simulink model "whole_system"  (R2016a)
settings: Solver=VariableStepAuto  StartTime=0.0  StopTime=0.25*100e6  RelTol=1e-3
libraries: xbsIndex_r4 x92, powerlib_meascontrol x4
settings Model: Creator=Jorge  LastModifiedBy=Jorge

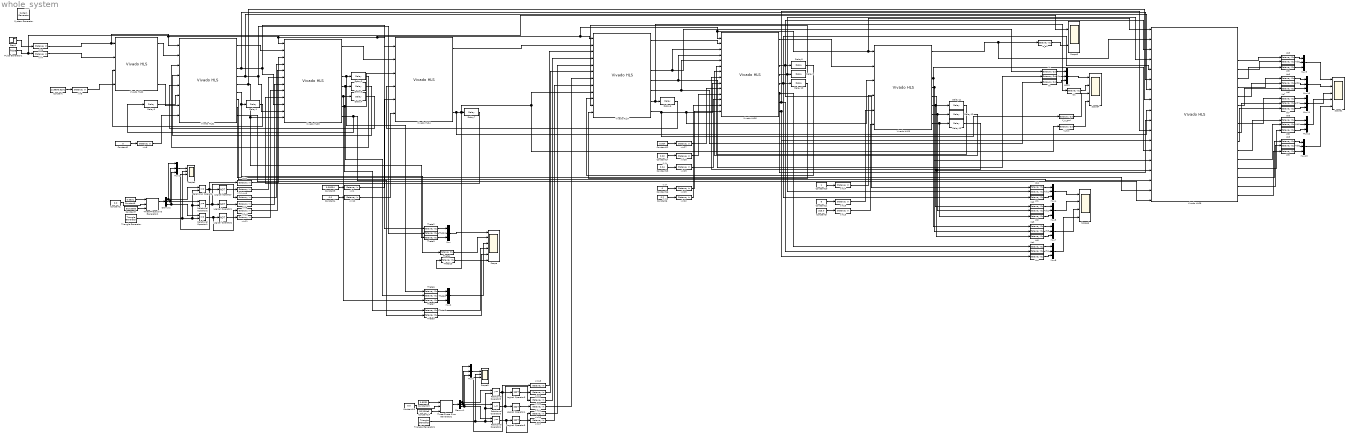
== system whole_system ==
  note: 0.04
  note: 0.04
  note: 0.04
  " System Generator" : xbsIndex_r4/ System Generator  Tag=genX  xilinxfamily=zynq  part=xc7z020  speed=-1  package=clg400  synthesis_tool=Vivado  clock_wrapper=Clock Enables  directory=./netlist  proj_type=Vivado  Synth_file=Vivado Synthesis Defaults  Impl_file=Vivado Implementation Defaults  testbench=off  simulink_period=1  sysclk_period=10  dcm_input_clock_period=10  incr_netlist=off  trim_vbits=Everywhere in SubSystem  dbl_ovrd=According to Block Masks  core_generation=According to Block Masks  run_coregen=off  deprecated_control=off  eval_field=0  block_type=sysgen
  Constant : Constant  Value=119856.8291
  Constant1 : Constant  Value=0.0
  Constant10 : Constant
  Constant11 : Constant  Value=8
  Constant12 : Constant  Value=0.004
  Constant13 : Constant  Value=0.0
  Constant14 : Constant  Value=50/100e6
  Constant16 : Constant  Value=0
  Constant17 : Constant  Value=0.02
  Constant18 : Constant  Value=0.04
  Constant19 : Constant  Value=0.6531
  Constant2 : Constant  Value=0
  Constant3 : Constant  Value=0.00004
  Constant4 : Constant  Value=0.0
  Constant5 : Constant  Value=325.0
  Constant6 : Constant  Value=0.5
  Constant7 : Constant  Value=50/100e6
  Constant8 : Constant  Value=0.6531
  Delay{1..13} (13 alike) : xbsIndex_r4/Delay  rst=off  infoeditControl=Selection of Reset will increase slice count due to use of real FFs and instead of SRLs  en=off  latency=1  reg_retiming=off  dbl_ovrd=off  block_type=delay
  Demux1 : Demux  Outputs=3
  Demux2 : Demux  Outputs=3
  Idc : xbsIndex_r4/Gateway Out  inherit_from_input=off  hdl_port=on  rows=1  columns=1  UseAsDAC=off  DACChannel='1'  interface=None  automatic_assignment=on  address_offset=hex2dec('00')  intf_name=''  intf_description=''  timing_constraint=None  locs_specified=off  LOCs={}  io_standard={}  block_type=gatewayout
  Is_a2 : xbsIndex_r4/Gateway Out  inherit_from_input=off  hdl_port=on  rows=1  columns=1  UseAsDAC=off  DACChannel='1'  interface=None  automatic_assignment=on  address_offset=hex2dec('00')  intf_name=''  intf_description=''  timing_constraint=None  locs_specified=off  LOCs={}  io_standard={}  block_type=gatewayout
  Logical Operator{,1..5} (6 alike) : Logic  Operator=NOT  AllPortsSameDT=off  OutDataTypeStr=boolean
  Mux{,1..13} (14 alike) : Mux  Inputs=3
  Pulse Generator1 : DiscretePulseGenerator  PulseType=Time based  Period=200  PulseWidth=50
  Relational Operator{,1..5} (6 alike) : RelationalOperator  OutDataTypeStr=boolean  ZeroCross=off
  Scope : Scope  NumInputPorts=6
  Scope1 : Scope  NumInputPorts=5
  Scope{2,4..6} (4 alike) : Scope  NumInputPorts=4
  Scope3 : Scope  NumInputPorts=2
  Step1 : Step  Time=1e-6  SampleTime=0
  Theta{1..10} (10 alike) : xbsIndex_r4/Gateway Out  inherit_from_input=off  hdl_port=on  rows=1  columns=1  UseAsDAC=off  DACChannel='1'  interface=None  automatic_assignment=on  address_offset=hex2dec('00')  intf_name=''  intf_description=''  timing_constraint=None  locs_specified=off  LOCs={}  io_standard={}  block_type=gatewayout
  Three-Phase Sine Generator1 : powerlib_meascontrol/Pulse & Signal Generators/Three-Phase Sine Generator  Ts=1
  Three-Phase Sine Generator2 : powerlib_meascontrol/Pulse & Signal Generators/Three-Phase Sine Generator  Ts=1
  Triangle Generator : powerlib_meascontrol/Pulse & Signal Generators/Triangle Generator  Freq=5e3/100e6  Phase=0  Ts=1
  Triangle Generator1 : powerlib_meascontrol/Pulse & Signal Generators/Triangle Generator  Freq=5e3/100e6  Phase=0  Ts=1
  V_bus : xbsIndex_r4/Gateway Out  inherit_from_input=off  hdl_port=on  rows=1  columns=1  UseAsDAC=off  DACChannel='1'  interface=None  automatic_assignment=on  address_offset=hex2dec('00')  intf_name=''  intf_description=''  timing_constraint=None  locs_specified=off  LOCs={}  io_standard={}  block_type=gatewayout
  V_n_gnd : xbsIndex_r4/Gateway Out  inherit_from_input=off  hdl_port=on  rows=1  columns=1  UseAsDAC=off  DACChannel='1'  interface=None  automatic_assignment=on  address_offset=hex2dec('00')  intf_name=''  intf_description=''  timing_constraint=None  locs_specified=off  LOCs={}  io_standard={}  block_type=gatewayout
  Va{,1..9} (10 alike) : xbsIndex_r4/Gateway Out  inherit_from_input=off  hdl_port=on  rows=1  columns=1  UseAsDAC=off  DACChannel='1'  interface=None  automatic_assignment=on  address_offset=hex2dec('00')  intf_name=''  intf_description=''  timing_constraint=None  locs_specified=off  LOCs={}  io_standard={}  block_type=gatewayout
  Vb{,1..9} (10 alike) : xbsIndex_r4/Gateway Out  inherit_from_input=off  hdl_port=on  rows=1  columns=1  UseAsDAC=off  DACChannel='1'  interface=None  automatic_assignment=on  address_offset=hex2dec('00')  intf_name=''  intf_description=''  timing_constraint=None  locs_specified=off  LOCs={}  io_standard={}  block_type=gatewayout
  Vc{,1..9} (10 alike) : xbsIndex_r4/Gateway Out  inherit_from_input=off  hdl_port=on  rows=1  columns=1  UseAsDAC=off  DACChannel='1'  interface=None  automatic_assignment=on  address_offset=hex2dec('00')  intf_name=''  intf_description=''  timing_constraint=None  locs_specified=off  LOCs={}  io_standard={}  block_type=gatewayout
  Vivado HLS1 : xbsIndex_r4/Vivado HLS  anytable='C:/Users/Jorge/Documents/GitHub/nvHIL/hls/pmsm_V2/pmsm_V2_prj/sol_sysgen'  fast_sim=off  display_datatype=on  rate_propagation_method=Simulink system period  model_file_path=''  latency=1  block_type=hls
      settings: infoedit=This block allows including C,C++ and SystemC source files in System Generator for DSP designs.
  Vivado HLS2 : xbsIndex_r4/Vivado HLS  anytable='C:\Users\Jorge\Documents\GitHub\nvHIL\hls\wind_tur_V2\wind_turb_V2_prj\sol_sysgen'  fast_sim=off  display_datatype=on  rate_propagation_method=Simulink system period  model_file_path=''  latency=1  block_type=hls
      settings: infoedit=This block allows including C,C++ and SystemC source files in System Generator for DSP designs.
  Vivado HLS3 : xbsIndex_r4/Vivado HLS  anytable='C:\Users\Jorge\Documents\GitHub\nvHIL\hls\pmsm_3ph_inv_V2\pmsm_inv_prj\sol_sysgen'  fast_sim=off  display_datatype=on  rate_propagation_method=Simulink system period  model_file_path=''  latency=1  block_type=hls
      settings: infoedit=This block allows including C,C++ and SystemC source files in System Generator for DSP designs.
  Vivado HLS4 : xbsIndex_r4/Vivado HLS  anytable='C:\Users\Jorge\Documents\GitHub\nvHIL\hls\DC_bus_V2\dc_bus_prj\sol_sysgen'  fast_sim=off  display_datatype=on  rate_propagation_method=Simulink system period  model_file_path=''  latency=1  block_type=hls
      settings: infoedit=This block allows including C,C++ and SystemC source files in System Generator for DSP designs.
  Vivado HLS5 : xbsIndex_r4/Vivado HLS  anytable='C:\Users\Jorge\Documents\GitHub\nvHIL\hls\grid_V2\grid_prj\sol_sysgen'  fast_sim=off  display_datatype=on  rate_propagation_method=Simulink system period  model_file_path=''  latency=1  block_type=hls
      settings: infoedit=This block allows including C,C++ and SystemC source files in System Generator for DSP designs.
  Vivado HLS6 : xbsIndex_r4/Vivado HLS  anytable='C:\Users\Jorge\Documents\GitHub\nvHIL\hls\LCL_filter_V2\LCL_filter_prj\sol_sysgen'  fast_sim=off  display_datatype=on  rate_propagation_method=Simulink system period  model_file_path=''  latency=1  block_type=hls
      settings: infoedit=This block allows including C,C++ and SystemC source files in System Generator for DSP designs.
  Vivado HLS7 : xbsIndex_r4/Vivado HLS  anytable='C:\Users\Jorge\Documents\GitHub\nvHIL\hls\grid_3ph_inv_V2\grid_3ph_bridge_prj\sol_sysgen'  fast_sim=off  display_datatype=on  rate_propagation_method=Simulink system period  model_file_path=''  latency=1  block_type=hls
      settings: infoedit=This block allows including C,C++ and SystemC source files in System Generator for DSP designs.
  Vivado HLS8 : xbsIndex_r4/Vivado HLS  anytable='C:\Users\Jorge\Documents\GitHub\nvHIL\hls\gain_offset_truncation_V2\gain_offset_truncation_prj\sol_sysgen'  fast_sim=off  display_datatype=on  rate_propagation_method=Simulink system period  model_file_path=''  latency=1  block_type=hls
      settings: infoedit=This block allows including C,C++ and SystemC source files in System Generator for DSP designs.
  xin1 : xbsIndex_r4/Gateway In  gui_display_data_type=Fixed-point  arith_type="Signed  (2's comp)"  n_bits=19  bin_pt=18  preci_type=Single  exp_width=8  frac_width=24  rows=1  columns=1  quantization="Round  (unbiased: +/- Inf)"  overflow=Saturate  period=1  UseAsADC=off  ADCChannel='1'  interface=None  automatic_assignment=on  address_offset=hex2dec('00')  intf_name=''  intf_description=''  default_value=0  timing_constraint=None  locs_specified=off  LOCs={}  io_standard={}  inherit_from_input=off  hdl_port=on  dbl_ovrd=off  block_type=gatewayin
  xin{2..4,9..11,16..21} (12 alike) : xbsIndex_r4/Gateway In  gui_display_data_type=Boolean  arith_type=Boolean  n_bits=18  bin_pt=6  preci_type=Single  exp_width=8  frac_width=24  rows=1  columns=1  quantization="Round  (unbiased: +/- Inf)"  overflow=Saturate  period=1  UseAsADC=off  ADCChannel='1'  interface=None  automatic_assignment=on  address_offset=hex2dec('00')  intf_name=''  intf_description=''  default_value=0  timing_constraint=None  locs_specified=off  LOCs={}  io_standard={}  inherit_from_input=off  hdl_port=on  dbl_ovrd=off  block_type=gatewayin
  xin12 : xbsIndex_r4/Gateway In  gui_display_data_type=Fixed-point  arith_type="Signed  (2's comp)"  n_bits=2  bin_pt=1  preci_type=Single  exp_width=8  frac_width=24  rows=1  columns=1  quantization="Round  (unbiased: +/- Inf)"  overflow=Saturate  period=1  UseAsADC=off  ADCChannel='1'  interface=None  automatic_assignment=on  address_offset=hex2dec('00')  intf_name=''  intf_description=''  default_value=0  timing_constraint=None  locs_specified=off  LOCs={}  io_standard={}  inherit_from_input=off  hdl_port=on  dbl_ovrd=off  block_type=gatewayin
  xin13 : xbsIndex_r4/Gateway In  gui_display_data_type=Fixed-point  arith_type="Signed  (2's comp)"  n_bits=25  bin_pt=9  preci_type=Single  exp_width=8  frac_width=24  rows=1  columns=1  quantization="Round  (unbiased: +/- Inf)"  overflow=Saturate  period=1  UseAsADC=off  ADCChannel='1'  interface=None  automatic_assignment=on  address_offset=hex2dec('00')  intf_name=''  intf_description=''  default_value=0  timing_constraint=None  locs_specified=off  LOCs={}  io_standard={}  inherit_from_input=off  hdl_port=on  dbl_ovrd=off  block_type=gatewayin
  xin14 : xbsIndex_r4/Gateway In  gui_display_data_type=Boolean  arith_type=Boolean  n_bits=2  bin_pt=1  preci_type=Single  exp_width=8  frac_width=24  rows=1  columns=1  quantization="Round  (unbiased: +/- Inf)"  overflow=Saturate  period=1  UseAsADC=off  ADCChannel='1'  interface=None  automatic_assignment=on  address_offset=hex2dec('00')  intf_name=''  intf_description=''  default_value=0  timing_constraint=None  locs_specified=off  LOCs={}  io_standard={}  inherit_from_input=off  hdl_port=on  dbl_ovrd=off  block_type=gatewayin
  xin15 : xbsIndex_r4/Gateway In  gui_display_data_type=Fixed-point  arith_type="Signed  (2's comp)"  n_bits=16  bin_pt=1  preci_type=Single  exp_width=8  frac_width=24  rows=1  columns=1  quantization="Round  (unbiased: +/- Inf)"  overflow=Saturate  period=1  UseAsADC=off  ADCChannel='1'  interface=None  automatic_assignment=on  address_offset=hex2dec('00')  intf_name=''  intf_description=''  default_value=0  timing_constraint=None  locs_specified=off  LOCs={}  io_standard={}  inherit_from_input=off  hdl_port=on  dbl_ovrd=off  block_type=gatewayin
  xin22 : xbsIndex_r4/Gateway In  gui_display_data_type=Fixed-point  arith_type="Signed  (2's comp)"  n_bits=16  bin_pt=13  preci_type=Single  exp_width=8  frac_width=24  rows=1  columns=1  quantization="Round  (unbiased: +/- Inf)"  overflow=Saturate  period=1  UseAsADC=off  ADCChannel='1'  interface=None  automatic_assignment=on  address_offset=hex2dec('00')  intf_name=''  intf_description=''  default_value=0  timing_constraint=None  locs_specified=off  LOCs={}  io_standard={}  inherit_from_input=off  hdl_port=on  dbl_ovrd=off  block_type=gatewayin
  xin25 : xbsIndex_r4/Gateway In  gui_display_data_type=Boolean  arith_type=Boolean  n_bits=16  bin_pt=15  preci_type=Single  exp_width=8  frac_width=24  rows=1  columns=1  quantization="Round  (unbiased: +/- Inf)"  overflow=Saturate  period=1  UseAsADC=off  ADCChannel='1'  interface=None  automatic_assignment=on  address_offset=hex2dec('00')  intf_name=''  intf_description=''  default_value=0  timing_constraint=None  locs_specified=off  LOCs={}  io_standard={}  inherit_from_input=off  hdl_port=on  dbl_ovrd=off  block_type=gatewayin
  xin27 : xbsIndex_r4/Gateway In  gui_display_data_type=Fixed-point  arith_type="Signed  (2's comp)"  n_bits=16  bin_pt=15  preci_type=Single  exp_width=8  frac_width=24  rows=1  columns=1  quantization="Round  (unbiased: +/- Inf)"  overflow=Saturate  period=1  UseAsADC=off  ADCChannel='1'  interface=None  automatic_assignment=on  address_offset=hex2dec('00')  intf_name=''  intf_description=''  default_value=0  timing_constraint=None  locs_specified=off  LOCs={}  io_standard={}  inherit_from_input=off  hdl_port=on  dbl_ovrd=off  block_type=gatewayin
  xin28 : xbsIndex_r4/Gateway In  gui_display_data_type=Fixed-point  arith_type="Signed  (2's comp)"  n_bits=16  bin_pt=15  preci_type=Single  exp_width=8  frac_width=24  rows=1  columns=1  quantization="Round  (unbiased: +/- Inf)"  overflow=Saturate  period=1  UseAsADC=off  ADCChannel='1'  interface=None  automatic_assignment=on  address_offset=hex2dec('00')  intf_name=''  intf_description=''  default_value=0  timing_constraint=None  locs_specified=off  LOCs={}  io_standard={}  inherit_from_input=off  hdl_port=on  dbl_ovrd=off  block_type=gatewayin
  xin29 : xbsIndex_r4/Gateway In  gui_display_data_type=Fixed-point  arith_type="Signed  (2's comp)"  n_bits=16  bin_pt=15  preci_type=Single  exp_width=8  frac_width=24  rows=1  columns=1  quantization="Round  (unbiased: +/- Inf)"  overflow=Saturate  period=1  UseAsADC=off  ADCChannel='1'  interface=None  automatic_assignment=on  address_offset=hex2dec('00')  intf_name=''  intf_description=''  default_value=0  timing_constraint=None  locs_specified=off  LOCs={}  io_standard={}  inherit_from_input=off  hdl_port=on  dbl_ovrd=off  block_type=gatewayin
  xin5 : xbsIndex_r4/Gateway In  gui_display_data_type=Fixed-point  arith_type="Signed  (2's comp)"  n_bits=21  bin_pt=1  preci_type=Single  exp_width=8  frac_width=24  rows=1  columns=1  quantization="Round  (unbiased: +/- Inf)"  overflow=Saturate  period=1  UseAsADC=off  ADCChannel='1'  interface=None  automatic_assignment=on  address_offset=hex2dec('00')  intf_name=''  intf_description=''  default_value=0  timing_constraint=None  locs_specified=off  LOCs={}  io_standard={}  inherit_from_input=off  hdl_port=on  dbl_ovrd=off  block_type=gatewayin
  xin6 : xbsIndex_r4/Gateway In  gui_display_data_type=Boolean  arith_type=Boolean  n_bits=16  bin_pt=10  preci_type=Single  exp_width=8  frac_width=24  rows=1  columns=1  quantization="Round  (unbiased: +/- Inf)"  overflow=Saturate  period=1  UseAsADC=off  ADCChannel='1'  interface=None  automatic_assignment=on  address_offset=hex2dec('00')  intf_name=''  intf_description=''  default_value=0  timing_constraint=None  locs_specified=off  LOCs={}  io_standard={}  inherit_from_input=off  hdl_port=on  dbl_ovrd=off  block_type=gatewayin
  xin7 : xbsIndex_r4/Gateway In  gui_display_data_type=Boolean  arith_type=Boolean  n_bits=16  bin_pt=10  preci_type=Single  exp_width=8  frac_width=24  rows=1  columns=1  quantization="Round  (unbiased: +/- Inf)"  overflow=Saturate  period=1  UseAsADC=off  ADCChannel='1'  interface=None  automatic_assignment=on  address_offset=hex2dec('00')  intf_name=''  intf_description=''  default_value=0  timing_constraint=None  locs_specified=off  LOCs={}  io_standard={}  inherit_from_input=off  hdl_port=on  dbl_ovrd=off  block_type=gatewayin
  xin8 : xbsIndex_r4/Gateway In  gui_display_data_type=Boolean  arith_type=Boolean  n_bits=21  bin_pt=1  preci_type=Single  exp_width=8  frac_width=24  rows=1  columns=1  quantization="Round  (unbiased: +/- Inf)"  overflow=Saturate  period=1  UseAsADC=off  ADCChannel='1'  interface=None  automatic_assignment=on  address_offset=hex2dec('00')  intf_name=''  intf_description=''  default_value=0  timing_constraint=None  locs_specified=off  LOCs={}  io_standard={}  inherit_from_input=off  hdl_port=on  dbl_ovrd=off  block_type=gatewayin
  wires:
  Step1/1 -> xin6/1
  Pulse Generator1/1 -> Scope3/1, xin7/1
  Constant/1 -> xin5/1
  Theta4/1 -> Scope/2
  xin6/1 -> Vivado HLS1/1, Vivado HLS3/1, Vivado HLS8/1, Vivado HLS5/1, Vivado HLS6/1, Vivado HLS7/1, Vivado HLS4/1, Vivado HLS2/1
  xin7/1 -> Vivado HLS2/2
  Vivado HLS2/1 -> Vivado HLS1/2
  Vivado HLS2/4 -> Vivado HLS1/7
  Delay1/1 -> Vivado HLS2/3
  xin5/1 -> Vivado HLS2/4
  Demux2/1 -> Mux1/1, Relational Operator/1
  Demux2/2 -> Mux1/2, Relational Operator2/1
  Demux2/3 -> Mux1/3, Relational Operator1/1
  Triangle Generator/1 -> Scope2/2, Relational Operator1/2, Relational Operator2/2, Relational Operator/2
  Relational Operator/1 -> xin2/1, Logical Operator/1, Scope2/3
  Constant7/1 -> Three-Phase Sine Generator1/3
  Constant8/1 -> Three-Phase Sine Generator1/1
  Three-Phase Sine Generator1/1 -> Demux2/1
  Mux1/1 -> Scope2/1
  Constant1/1 -> Three-Phase Sine Generator1/2
  Mux/1 -> Scope/1
  Theta2/1 -> Mux/1
  Theta1/1 -> Mux/2
  Theta3/1 -> Mux/3
  Vivado HLS1/7 -> Theta4/1, Delay1/1
  Vivado HLS1/1 -> Vivado HLS3/2
  Vivado HLS1/4 -> Vivado HLS8/6, Theta2/1, Vivado HLS3/10
  Vivado HLS1/5 -> Vivado HLS8/7, Theta1/1, Vivado HLS3/11
  Vivado HLS1/6 -> Vivado HLS8/8, Theta3/1, Vivado HLS3/12
  Vivado HLS3/4 -> Theta6/1, Delay2/1
  Vivado HLS3/5 -> Theta5/1, Delay3/1
  Vivado HLS3/6 -> Theta7/1, Delay4/1
  Delay2/1 -> Vivado HLS1/3
  Delay3/1 -> Vivado HLS1/4
  Delay4/1 -> Vivado HLS1/5
  Theta6/1 -> Mux2/1
  Theta5/1 -> Mux2/2
  Theta7/1 -> Mux2/3
  Mux2/1 -> Scope/3
  Vivado HLS3/8 -> Delay5/1, Theta9/1
  Theta8/1 -> Scope/4
  Theta9/1 -> Scope/5
  Delay5/1 -> Vivado HLS1/6
  Relational Operator1/1 -> xin10/1, Logical Operator2/1
  Relational Operator2/1 -> xin4/1, Logical Operator1/1
  Logical Operator2/1 -> xin11/1
  Logical Operator1/1 -> xin9/1
  Logical Operator/1 -> xin3/1
  xin2/1 -> Vivado HLS3/3
  xin4/1 -> Vivado HLS3/4
  xin10/1 -> Vivado HLS3/5
  xin3/1 -> Vivado HLS3/6
  xin9/1 -> Vivado HLS3/7
  xin11/1 -> Vivado HLS3/8
  Vivado HLS3/1 -> Vivado HLS4/2
  Vivado HLS3/7 -> Vivado HLS4/3, Theta8/1
  Constant3/1 -> xin1/1
  xin1/1 -> Vivado HLS4/5
  Constant4/1 -> xin12/1
  xin12/1 -> Vivado HLS4/6
  ? -> ?
  Theta10/1 -> Scope/6
  Delay7/1 -> Vivado HLS3/9
  Is_a2/1 -> Scope3/2
  Va/1 -> Mux3/1
  Vb/1 -> Mux3/2
  Vc/1 -> Mux3/3
  Demux1/1 -> Mux6/1, Relational Operator3/1
  Demux1/2 -> Mux6/2, Relational Operator5/1
  Demux1/3 -> Mux6/3, Relational Operator4/1
  Triangle Generator1/1 -> Scope5/2, Relational Operator4/2, Relational Operator5/2, Relational Operator3/2
  Relational Operator3/1 -> xin18/1, Logical Operator3/1, Scope5/3
  Constant14/1 -> Three-Phase Sine Generator2/3
  Constant19/1 -> Three-Phase Sine Generator2/1
  Three-Phase Sine Generator2/1 -> Demux1/1
  Mux6/1 -> Scope5/1
  Constant13/1 -> Three-Phase Sine Generator2/2
  Relational Operator4/1 -> xin16/1, Logical Operator5/1
  Relational Operator5/1 -> xin20/1, Logical Operator4/1
  Logical Operator5/1 -> xin17/1
  Logical Operator4/1 -> xin21/1
  Logical Operator3/1 -> xin19/1
  Vivado HLS4/4 -> Vivado HLS8/9, Vivado HLS7/9, V_bus/1, Theta10/1, Delay7/1
  Vivado HLS7/7 -> Idc/1, Delay6/1
  Vivado HLS6/4 -> Vivado HLS8/3, Va1/1, Delay8/1
  Vivado HLS6/5 -> Vb1/1, Vivado HLS8/4, Delay9/1
  Vivado HLS6/6 -> Vivado HLS8/5, Vc1/1, Delay10/1
  Constant12/1 -> xin27/1
  Constant17/1 -> xin28/1
  Constant18/1 -> xin29/1
  xin27/1 -> Vivado HLS6/10
  xin28/1 -> Vivado HLS6/11
  xin29/1 -> Vivado HLS6/12
  Vivado HLS7/8 -> Vivado HLS5/3, Vivado HLS6/9, V_n_gnd/1
  Constant10/1 -> xin14/1
  xin14/1 -> Vivado HLS5/4
  Constant11/1 -> xin15/1
  xin15/1 -> Vivado HLS5/5
  Vivado HLS5/1 -> Vivado HLS8/2, Is_a2/1
  Vivado HLS5/9 -> Vc2/1, Delay13/1
  Vivado HLS5/8 -> Vb2/1, Delay12/1
  Vivado HLS5/7 -> Va2/1, Delay11/1
  Vivado HLS7/4 -> Vivado HLS6/3, Va/1
  Vivado HLS7/5 -> Vivado HLS6/4, Vb/1
  Vivado HLS7/6 -> Vivado HLS6/5, Vc/1
  Mux3/1 -> Scope4/1
  Idc/1 -> Scope4/2
  V_n_gnd/1 -> Scope4/3
  V_bus/1 -> Scope4/4
  xin18/1 -> Vivado HLS7/3
  xin20/1 -> Vivado HLS7/4
  xin16/1 -> Vivado HLS7/5
  xin19/1 -> Vivado HLS7/6
  xin21/1 -> Vivado HLS7/7
  xin17/1 -> Vivado HLS7/8
  Vivado HLS7/1 -> Vivado HLS6/2
  Vivado HLS6/1 -> Vivado HLS5/2
  Delay11/1 -> Vivado HLS6/6
  Delay12/1 -> Vivado HLS6/7
  Delay13/1 -> Vivado HLS6/8
  Va1/1 -> Mux4/1
  Vb1/1 -> Mux4/2
  Vc1/1 -> Mux4/3
  Mux4/1 -> Scope6/1
  Va2/1 -> Mux5/1
  Vb2/1 -> Mux5/2
  Vc2/1 -> Mux5/3
  Mux5/1 -> Scope6/2
  Delay8/1 -> Vivado HLS7/10
  Delay9/1 -> Vivado HLS7/11
  Delay10/1 -> Vivado HLS7/12
  Va3/1 -> Mux7/1
  Vb3/1 -> Mux7/2
  Vc3/1 -> Mux7/3
  Mux7/1 -> Scope6/3
  Vivado HLS5/4 -> Va3/1, Vivado HLS8/13
  Vivado HLS5/5 -> Vivado HLS8/14, Vb3/1
  Vivado HLS5/6 -> Vivado HLS8/15, Vc3/1
  Va4/1 -> Mux8/1
  Vb4/1 -> Mux8/2
  Vc4/1 -> Mux8/3
  Mux8/1 -> Scope6/4
  Vivado HLS6/7 -> Vivado HLS8/10, Va4/1
  Vivado HLS6/8 -> Vivado HLS8/11, Vb4/1
  Vivado HLS6/9 -> Vivado HLS8/12, Vc4/1
  Constant16/1 -> xin25/1
  Vivado HLS4/1 -> Vivado HLS7/2
  Delay6/1 -> Vivado HLS4/4
  Constant2/1 -> xin8/1
  xin8/1 -> Vivado HLS1/8
  Constant5/1 -> xin13/1
  xin13/1 -> Vivado HLS5/6
  xin25/1 -> Vivado HLS6/14
  Constant6/1 -> xin22/1
  xin22/1 -> Vivado HLS6/13
  Vivado HLS1/8 -> Vivado HLS8/16
  Vivado HLS1/9 -> Vivado HLS8/17
  Vivado HLS1/10 -> Vivado HLS8/18
  Vivado HLS8/4 -> Va5/1
  Vivado HLS8/5 -> Vb5/1
  Vivado HLS8/6 -> Vc5/1
  Vivado HLS8/7 -> Va6/1
  Vivado HLS8/8 -> Vb6/1
  Vivado HLS8/9 -> Vc6/1
  Vivado HLS8/11 -> Va7/1
  Vivado HLS8/12 -> Vb7/1
  Vivado HLS8/13 -> Vc7/1
  Vivado HLS8/14 -> Va8/1
  Vivado HLS8/15 -> Vb8/1
  Vivado HLS8/16 -> Vc8/1
  Vivado HLS8/17 -> Va9/1
  Vivado HLS8/18 -> Vb9/1
  Vivado HLS8/19 -> Vc9/1
  Vc5/1 -> Mux9/3
  Vb5/1 -> Mux9/2
  Va5/1 -> Mux9/1
  Vc6/1 -> Mux10/3
  Vb6/1 -> Mux10/2
  Va6/1 -> Mux10/1
  Vc7/1 -> Mux11/3
  Vb7/1 -> Mux11/2
  Va7/1 -> Mux11/1
  Va8/1 -> Mux12/1
  Vb8/1 -> Mux12/2
  Vc8/1 -> Mux12/3
  Va9/1 -> Mux13/1
  Vb9/1 -> Mux13/2
  Vc9/1 -> Mux13/3
  Mux13/1 -> Scope1/5
  Mux12/1 -> Scope1/4
  Mux11/1 -> Scope1/3
  Mux10/1 -> Scope1/2
  Mux9/1 -> Scope1/1
